simulink model "calcKalmanEstimate_th"  (R2022a)
settings: Solver=FixedStepAuto  StartTime=0.0  StopTime=algFinTime*60  FixedStep=kfgp.kfgpTimeStep*60/2  RelTol=1e-3
libraries: simulink x1, calcKalmanEstimate_ul x1
settings Model: Creator=Ayaz  LastModifiedBy=lhill8
settings SolverCC: AlgebraicLoopSolver=TrustRegion
settings DebuggingCC: UnconnectedInputMsg=warning  UnconnectedOutputMsg=warning  UnconnectedLineMsg=warning  SFMachineParentedDataDiag=warning

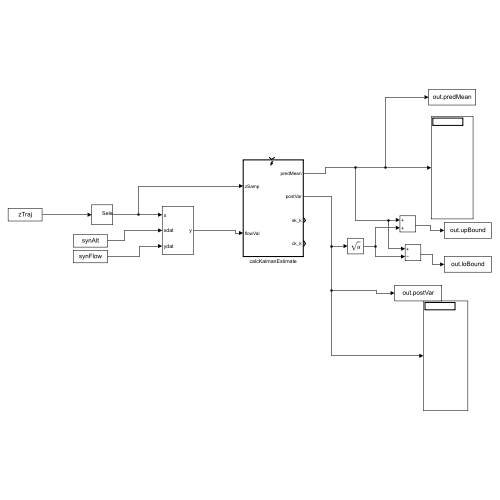
[thumbnail: Simulink's stored preview of the top-level diagram]
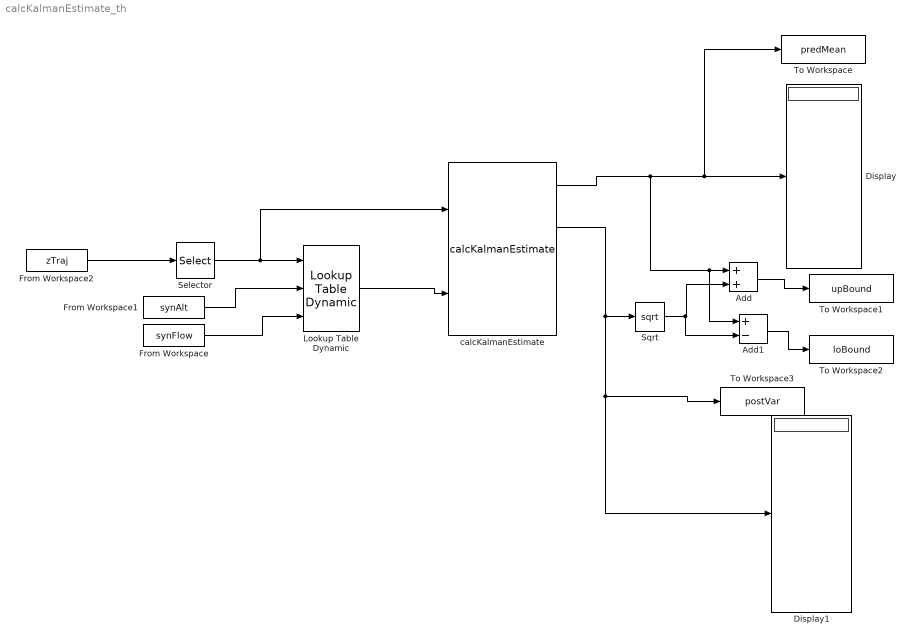
== system calcKalmanEstimate_th ==
  Add : Sum
  Add1 : Sum  Inputs=+-
  Display : Display
  Display1 : Display
  From Workspace : FromWorkspace  VariableName=synFlow
  From Workspace1 : FromWorkspace  VariableName=synAlt
  From Workspace2 : FromWorkspace  VariableName=zTraj
  Lookup Table Dynamic : simulink/Lookup Tables/Lookup Table Dynamic  LookUpMeth=Interpolation-Use End Values  OutDataType=fixdt('double')  OutScaling=[]  OutputDataTypeScalingMode=Specify via dialog  OutDataTypeStr=double  DoSatur=off
  Selector : Selector  InputPortWidth=2  IndexOptions=Index vector (dialog)  Indices=1  OutputSizes=1
  Sqrt : Sqrt
  To Workspace : ToWorkspace  VariableName=predMean  SaveFormat=Timeseries  SampleTime=-1
  To Workspace1 : ToWorkspace  VariableName=upBound  SaveFormat=Timeseries  SampleTime=-1
  To Workspace2 : ToWorkspace  VariableName=loBound  SaveFormat=Timeseries  SampleTime=-1
  To Workspace3 : ToWorkspace  VariableName=postVar  SaveFormat=Timeseries  SampleTime=-1
  calcKalmanEstimate : calcKalmanEstimate_ul/calcKalmanEstimate  hiLvlCtrl=hiLvlCtrl
  wires:
  Lookup Table Dynamic/1 -> calcKalmanEstimate/2
  From Workspace1/1 -> Lookup Table Dynamic/2
  From Workspace/1 -> Lookup Table Dynamic/3
  calcKalmanEstimate/1 -> Add1/1, Add/1, To Workspace/1, Display/1
  calcKalmanEstimate/2 -> Sqrt/1, To Workspace3/1, Display1/1
  Selector/1 -> calcKalmanEstimate/1, Lookup Table Dynamic/1
  Sqrt/1 -> Add1/2, Add/2
  Add/1 -> To Workspace1/1
  Add1/1 -> To Workspace2/1
  From Workspace2/1 -> Selector/1
